simulink model "Energy_Flow_Coordinator"  (R2016b)
settings: Solver=FixedStepDiscrete  StartTime=0.0  StopTime=inf  FixedStep=EgyFlowCoorr.tiSimnTiStep_C  RelTol=1e-3  EnableMultiTasking=on
undefined symbols (not defined in the file or in its folder): EgyFlowCoorr_swtAirCdnOptmr_INT, EgyFlowCoorr_swtCoolgSysOptmr_INT, EgyFlowCoorr_swtEgyFlowCoorrActv_INT, EgyFlowCoorr_swtElecSysOptmr_INT, EgyFlowCoorr_swtPnmSysOptmr_INT
settings Model: Creator=djuenema  LastModifiedBy=djuenema
settings DataIOCC: SaveFormat=StructureWithTime  SaveOutput=off  DSMLogging=off  VisualizeSimOutput=off  SaveTime=off  SignalLoggingName=Results
settings OptimizationCC: BlockReduction=off  ConditionallyExecuteInputs=off  LifeSpan=inf
settings DebuggingCC: AllowSymbolicDim=off  SFUnexpectedBacktrackingDiag=warning  SFNoUnconditionalDefaultTransitionDiag=warning  SFExecutionAtInitializationDiag=none
settings ModelReferenceCC: ModelReferenceNumInstancesAllowed=Single  PropagateSignalLabelsOutOfModel=off
settings GRTTargetCC: TargetLangStandard=C89/C90 (ANSI)
settings ConfigComp: CovMetricSettings=dw  CovHtmlReporting=on  CovSaveCumulativeToWorkspaceVar=on  CovSaveSingleToWorkspaceVar=on  CovExternalEMLEnable=off

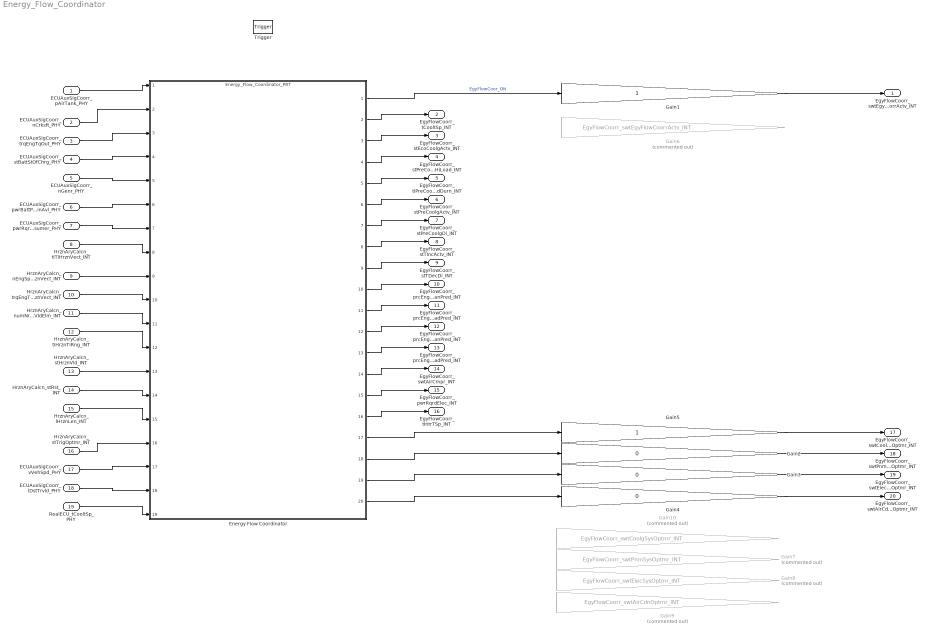
== system Energy_Flow_Coordinator ==
  ECUAuxSigCoorr_pAirTank_PHY : Inport
  ECUAuxSigCoorr_nCrksft_PHY : Inport  Port=2
  ECUAuxSigCoorr_trqEngTqOut_PHY : Inport  Port=3
  ECUAuxSigCoorr_stBattStOfChrg_PHY : Inport  Port=4
  ECUAuxSigCoorr_nGenr_PHY : Inport  Port=5
  ECUAuxSigCoorr_pwrBattPwrMinAvl_PHY : Inport  Port=6
  ECUAuxSigCoorr_pwrRqrdElecPwrConsumer_PHY : Inport  Port=7
  HrznAryCalcn_tiTiHrznVect_INT : Inport  Port=8
  HrznAryCalcn_nEngSpdHrznVect_INT : Inport  Port=9
  HrznAryCalcn_trqEngTqHrznVect_INT : Inport  Port=10
  HrznAryCalcn_numNrHrznVldElm_INT : Inport  Port=11
  HrznAryCalcn_tiHrznTiRng_INT : Inport  Port=12
  HrznAryCalcn_stHrznVld_INT : Inport  Port=13
  HrznAryCalcn_stRst_INT : Inport  Port=14
  HrznAryCalcn_lHrznLen_INT : Inport  Port=15
  HrznAryCalcn_stTrigOptmr_INT : Inport  Port=16
  ECUAuxSigCoorr_vVehSpd_PHY : Inport  Port=17
  ECUAuxSigCoorr_lDstTrvld_PHY : Inport  Port=18
  RealECU_tCooltSp_PHY : Inport  Port=19
  Trigger : TriggerPort  TriggerType=function-call  VariantControl=Variant  PortDimensions=1
  Energy Flow Coordinator : ModelReference  ModelNameDialog=Energy_Flow_Coordinator_PRT.slxp  ModelReferenceVersion=1.3  CopyOfModelProtected=on
  Gain1 : Gain  OutDataTypeStr=Inherit: Same as input  ParamDataTypeStr=Inherit: Same as input
  Gain10 : Gain  Commented=on  Gain=EgyFlowCoorr_swtCoolgSysOptmr_INT  OutDataTypeStr=Inherit: Same as input  ParamDataTypeStr=Inherit: Same as input
  Gain2 : Gain  Gain=0  OutDataTypeStr=Inherit: Same as input  ParamDataTypeStr=Inherit: Same as input
  Gain3 : Gain  Gain=0  OutDataTypeStr=Inherit: Same as input  ParamDataTypeStr=Inherit: Same as input
  Gain4 : Gain  Gain=0  OutDataTypeStr=Inherit: Same as input  ParamDataTypeStr=Inherit: Same as input
  Gain5 : Gain  OutDataTypeStr=Inherit: Same as input  ParamDataTypeStr=Inherit: Same as input
  Gain6 : Gain  Commented=on  Gain=EgyFlowCoorr_swtEgyFlowCoorrActv_INT  OutDataTypeStr=Inherit: Same as input  ParamDataTypeStr=Inherit: Same as input
  Gain7 : Gain  Commented=on  Gain=EgyFlowCoorr_swtPnmSysOptmr_INT  OutDataTypeStr=Inherit: Same as input  ParamDataTypeStr=Inherit: Same as input
  Gain8 : Gain  Commented=on  Gain=EgyFlowCoorr_swtElecSysOptmr_INT  OutDataTypeStr=Inherit: Same as input  ParamDataTypeStr=Inherit: Same as input
  Gain9 : Gain  Commented=on  Gain=EgyFlowCoorr_swtAirCdnOptmr_INT  OutDataTypeStr=Inherit: Same as input  ParamDataTypeStr=Inherit: Same as input
  EgyFlowCoorr_swtEgyFlowCoorrActv_INT : Outport
  EgyFlowCoorr_tCooltSp_INT : Outport  Port=2
  EgyFlowCoorr_stEcoCoolgActv_INT : Outport  Port=3
  EgyFlowCoorr_stPreCoolgHiLoad_INT : Outport  Port=4
  EgyFlowCoorr_tiPreCoolgHiLoadDurn_INT : Outport  Port=5
  EgyFlowCoorr_stPreCoolgActv_INT : Outport  Port=6
  EgyFlowCoorr_stPreCoolgDi_INT : Outport  Port=7
  EgyFlowCoorr_stTIncActv_INT : Outport  Port=8
  EgyFlowCoorr_stTDecDi_INT : Outport  Port=9
  EgyFlowCoorr_prcEngLoadFlMeanPred_INT : Outport  Port=10
  EgyFlowCoorr_prcEngLoadPred_INT : Outport  Port=11
  EgyFlowCoorr_prcEngDrgLoadFlMeanPred_INT : Outport  Port=12
  EgyFlowCoorr_prcEngDrgLoadPred_INT : Outport  Port=13
  EgyFlowCoorr_swtAirCmpr_INT : Outport  Port=14
  EgyFlowCoorr_pwrRqrdElec_INT : Outport  Port=15
  EgyFlowCoorr_tIntrTSp_INT : Outport  Port=16
  EgyFlowCoorr_swtCoolgSysOptmr_INT : Outport  Port=17
  EgyFlowCoorr_swtPnmSysOptmr_INT : Outport  Port=18
  EgyFlowCoorr_swtElecSysOptmr_INT : Outport  Port=19
  EgyFlowCoorr_swtAirCdnOptmr_INT : Outport  Port=20
  wires:
  ECUAuxSigCoorr_pAirTank_PHY/1 -> Energy Flow Coordinator/1
  Energy Flow Coordinator/1 -> Gain1/1  "EgyFlowCoor_ON"
  Energy Flow Coordinator/2 -> EgyFlowCoorr_tCooltSp_INT/1
  Energy Flow Coordinator/3 -> EgyFlowCoorr_stEcoCoolgActv_INT/1
  Energy Flow Coordinator/4 -> EgyFlowCoorr_stPreCoolgHiLoad_INT/1
  Energy Flow Coordinator/5 -> EgyFlowCoorr_tiPreCoolgHiLoadDurn_INT/1
  Energy Flow Coordinator/7 -> EgyFlowCoorr_stPreCoolgDi_INT/1
  Energy Flow Coordinator/8 -> EgyFlowCoorr_stTIncActv_INT/1
  Energy Flow Coordinator/6 -> EgyFlowCoorr_stPreCoolgActv_INT/1
  ECUAuxSigCoorr_trqEngTqOut_PHY/1 -> Energy Flow Coordinator/3
  ECUAuxSigCoorr_nCrksft_PHY/1 -> Energy Flow Coordinator/2
  Gain1/1 -> EgyFlowCoorr_swtEgyFlowCoorrActv_INT/1
  Energy Flow Coordinator/9 -> EgyFlowCoorr_stTDecDi_INT/1
  Energy Flow Coordinator/14 -> EgyFlowCoorr_swtAirCmpr_INT/1
  Energy Flow Coordinator/10 -> EgyFlowCoorr_prcEngLoadFlMeanPred_INT/1
  Energy Flow Coordinator/13 -> EgyFlowCoorr_prcEngDrgLoadPred_INT/1
  Energy Flow Coordinator/15 -> EgyFlowCoorr_pwrRqrdElec_INT/1
  Energy Flow Coordinator/11 -> EgyFlowCoorr_prcEngLoadPred_INT/1
  Energy Flow Coordinator/16 -> EgyFlowCoorr_tIntrTSp_INT/1
  Energy Flow Coordinator/12 -> EgyFlowCoorr_prcEngDrgLoadFlMeanPred_INT/1
  ECUAuxSigCoorr_stBattStOfChrg_PHY/1 -> Energy Flow Coordinator/4
  ECUAuxSigCoorr_nGenr_PHY/1 -> Energy Flow Coordinator/5
  ECUAuxSigCoorr_pwrRqrdElecPwrConsumer_PHY/1 -> Energy Flow Coordinator/7
  ECUAuxSigCoorr_pwrBattPwrMinAvl_PHY/1 -> Energy Flow Coordinator/6
  Energy Flow Coordinator/17 -> Gain5/1
  Energy Flow Coordinator/18 -> Gain2/1
  Energy Flow Coordinator/19 -> Gain3/1
  Energy Flow Coordinator/20 -> Gain4/1
  HrznAryCalcn_tiTiHrznVect_INT/1 -> Energy Flow Coordinator/8
  HrznAryCalcn_trqEngTqHrznVect_INT/1 -> Energy Flow Coordinator/10
  HrznAryCalcn_nEngSpdHrznVect_INT/1 -> Energy Flow Coordinator/9
  HrznAryCalcn_numNrHrznVldElm_INT/1 -> Energy Flow Coordinator/11
  HrznAryCalcn_tiHrznTiRng_INT/1 -> Energy Flow Coordinator/12
  HrznAryCalcn_stRst_INT/1 -> Energy Flow Coordinator/14
  HrznAryCalcn_stHrznVld_INT/1 -> Energy Flow Coordinator/13
  HrznAryCalcn_stTrigOptmr_INT/1 -> Energy Flow Coordinator/16
  ECUAuxSigCoorr_vVehSpd_PHY/1 -> Energy Flow Coordinator/17
  ECUAuxSigCoorr_lDstTrvld_PHY/1 -> Energy Flow Coordinator/18
  RealECU_tCooltSp_PHY/1 -> Energy Flow Coordinator/19
  HrznAryCalcn_lHrznLen_INT/1 -> Energy Flow Coordinator/15
  Gain5/1 -> EgyFlowCoorr_swtCoolgSysOptmr_INT/1
  Gain2/1 -> EgyFlowCoorr_swtPnmSysOptmr_INT/1
  Gain3/1 -> EgyFlowCoorr_swtElecSysOptmr_INT/1
  Gain4/1 -> EgyFlowCoorr_swtAirCdnOptmr_INT/1
